simulink model "physics_model"  (R2025b)
settings: Solver=VariableStepAuto  StartTime=0.0  StopTime=10.0  RelTol=1e-3
settings Model: Creator=samue  LastModifiedBy=samue

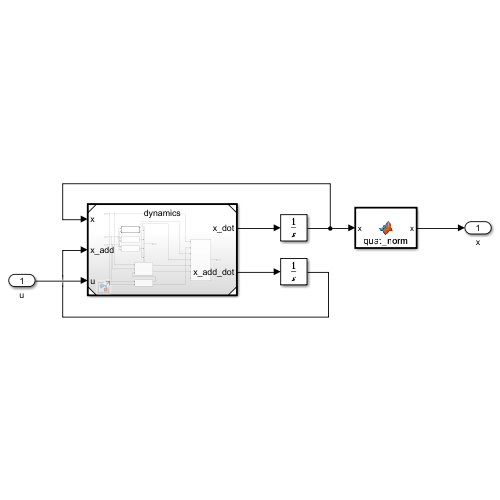
[thumbnail: Simulink's stored preview of the top-level diagram]
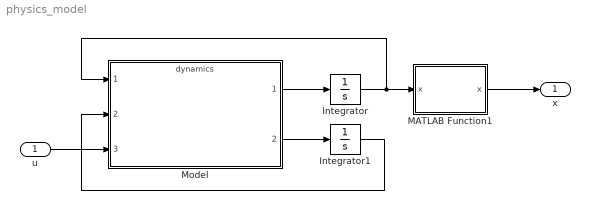
== system physics_model ==
  u : Inport
  Integrator : Integrator
  Integrator1 : Integrator
  MATLAB Function1 : MATLAB Function  TreatAsAtomicUnit=on
  Model : ModelReference  ModelNameDialog=dynamics.slx  SimulationMode=Normal  ModelReferenceVersion=1.20
  x : Outport
  wires:
  u/1 -> Model/3
  Model/2 -> Integrator1/1
  Model/1 -> Integrator/1
  Integrator1/1 -> Model/2
  Integrator/1 -> Model/1, MATLAB Function1/1("x ")
  MATLAB Function1/1(x) -> x/1

== matlab function physics_model/MATLAB Function1 ==
  data: x input; x output
function x = quat_norm(x)
% Normalises quaternoins to move back onto manifold
    q = x(7:10);
    x(7:10) = q / norm(q);
end
